simulink model "benchlink"  (R2024b)
settings: Solver=FixedStepDiscrete  StartTime=0.0  StopTime=0.005*16  RelTol=1e-3
model workspace (MAT data in the model file):
  socvcb : containers.Map (value not decoded)
values from neighbouring files (symbols this model uses):
  access = [32 0 4 36 32 0 4 36 32 0 4 36 ... (16 elements, 16x1)]    [all_variables.mat]
  qam_params =     [all_variables.mat]
undefined symbols (not defined in the file or in its folder): Add, j, QAM, rms, Shift
libraries: hdlsllib x53, simulink_need_slupdate x22, simulink x18, dspsigops x16, commdigbbndam3 x6, dsphdlmathfun2 x2, commchan3 x1, commrflib2 x1, dsphdlsigops2 x1, dspstat3 x1, dsphdlfiltering2 x1, simulink_extras x1
(part 5 of 5)

== matlab function benchlink/HDL_64QAM/HDLRxIPCore/QAM Rx HDL/Payload Delimiter/MATLAB Function1 ==
  data: isValid output; enable input; count input; isAccess output; qam_params parameter; accessChipStart input; packetSymLen input
function [isValid, isAccess] = ChipSync(enable, count, qam_params, accessChipStart, packetSymLen)
%#codegen

persistent state;
persistent counter;
%persistent packetLenInChips; % Renamed for clarity
persistent accessLen;

if isempty(state)
    state = false;
    counter = uint16(0);
    accessLen = uint16(qam_params.longTrainingChipLength);
end


packetLenInChips = uint16(packetSymLen * qam_params.spreadingFactor); 
isCountInRange = (mod(count, accessChipStart) < accessLen);


isCounterValid = (counter <= packetLenInChips) && (counter ~= 0);


isAccess = isCountInRange && isCounterValid;

if (counter <= packetLenInChips) && (counter ~= 0)
    isValid = true;
else
    isValid = false;
end
%%%%%%%%%%%%%%%%%%%%

% Internal logic using 'dvalid' (not an output) and decrementing counter
if state == false
    dvalid = false; % Not used as output
else % state == true
    dvalid = true;  % Not used as output
    % Decrement counter only when state is true
    if counter > 0
        counter = counter - 1;
    end
end

% state transition logic
if state == false && enable == true
    % Transition from false to true when enabled
    state = true;
    counter = packetLenInChips; % Use the pre-calculated value
elseif state == true && counter == 0
    % When state is true and counter reaches zero
    if enable == true
        % If still enabled, stay true and reset counter
        state = true;
        counter = packetLenInChips; % Use the pre-calculated value
    else
        % If not enabled when counter hits zero, transition back to false
        state = false;
        % Counter remains 0 until next enable
    end
end
% Implicit cases remain the same

end % End of function ChipSync

== matlab function benchlink/HDL_64QAM/HDLRxIPCore/QAM Rx HDL/EB Downsampler by 6_Old2/Chip Synchronization ==
  data: offset1 input; portSelect output; offset2 input; offset3 input; offset4 input; offset5 input; offset6 input
function portSelect  = chipSync(offset1, offset2, offset3, offset4, offset5, offset6)

[~,y] = max([offset1, offset2, offset3, offset4, offset5, offset6]);
portSelect = uint8(y);

== matlab function benchlink/HDL_64QAM/HDLRxIPCore/QAM Rx HDL/Payload Delimiter/Normalized Modulus/KeepMax ==
  data: in input; out output; qam_params parameter
function out  = keepMax(in, qam_params)

persistent x counter frameLen

if isempty(x)
    x = fi(0,1,18,15);
    counter    = uint16(0);
    frameLen = uint16((qam_params.packetSymLength*qam_params.spreadingFactor+...
        qam_params.preambleSymLength)*qam_params.Upsampling);
end

if (counter ~= 0)
    x = max(x,in);
    out = fi(x,1,18,15);
    counter = counter - 1;
else
    if (x > 5*in)
         out = fi(x,1,18,15);
         counter = frameLen;
    else
        x = fi(in,1,18,15);
        out = fi(x,1,18,15);
        counter = frameLen;
    end
end

== matlab function benchlink/HDL_64QAM/HDLRxIPCore/QAM Rx HDL/MF Filtering and Despreading/BER/ Integrate and Dump ==
  data: dValid input; validOut output; symbolIn input; sumOut output
function [validOut, sumOut] = intDump(dValid, symbolIn)
%#codegen

persistent sum_so_far counter

sumOut = fi(complex(0,0),1,18,13);
if isempty(sum_so_far)
sum_so_far = fi(complex(0,0),1,18,13);
end
validOut = false;
if isempty(counter)
counter = uint8(0);
end

if dValid
sum_so_far = fi(sum([sum_so_far symbolIn]),1,18,13);
counter = counter + 1;
end

if counter == 8
    sumOut = sum_so_far;
    validOut = true;
    counter = uint8(0);
    sum_so_far = fi(complex(0,0),1,18,13);
end

end

== matlab function benchlink/HDL_64QAM/HDLRxIPCore/QAM Rx HDL/MF Filtering and Despreading/BER/ Integrate and Dump1 ==
  data: dValid input; validOut output; symbolIn input; sumOut output
function [validOut, sumOut] = intDump(dValid, symbolIn)
%#codegen

persistent sum_so_far counter

sumOut = fi(complex(0,0),1,18,13);
if isempty(sum_so_far)
sum_so_far = fi(complex(0,0),1,18,13);
end
validOut = false;
if isempty(counter)
counter = uint8(0);
end

if dValid
sum_so_far = fi(sum([sum_so_far symbolIn]),1,18,13);
counter = counter + 1;
end

if counter == 8
    sumOut = sum_so_far;
    validOut = true;
    counter = uint8(0);
    sum_so_far = fi(complex(0,0),1,18,13);
end

end

== matlab function benchlink/HDL_64QAM/HDLRxIPCore/QAM Rx HDL/MF Filtering and Despreading/BER/BER Avg/MATLAB Function1 ==
  data: BERIn input; BERSumOut output; enable input; vecFullOut output; countOut output
function [BERSumOut, vecFullOut, countOut] = avgcodeVec(BERIn,enable)

persistent counter currVec fullVec isVecFull 

avgFactor = 8;

if isempty(counter)
    counter = uint8(0);
    currVec = ufi(0,19,9);
    fullVec = ufi(zeros(avgFactor,1),19,9);
    isVecFull = false;
end

if enable
    counter = counter + 1;
    fullVec(counter,:) = ufi(BERIn,19,9);
    if ~isVecFull
    currVec = ufi((currVec + BERIn),19,9);
    end
end

if isVecFull
    BERSumOut = ufi(sum(fullVec),19,9);
else
    BERSumOut = currVec;
end
countOut = counter;

if (counter == avgFactor)
        isVecFull = true;
        counter = uint8(0);
end
    
vecFullOut = isVecFull;

== matlab function benchlink/HDL_64QAM/HDLTxIPCore/QAMTxHDL/Controller FSM1 ==
  data: valid output; reset_preamble output; load_preamble output; load_data output; transmitNow input; packetsPerBurst input
function [valid, reset_preamble, load_preamble, load_data] = ControllerFSM(transmitNow,packetsPerBurst)
%#codegen
persistent packState stateCounter subDivCounter EoF txRequest 
%persistent packsIterate;
sType = numerictype(0,2,0);
cType = numerictype(0,16,0);
subDivType = numerictype(0,3,0); % Enough to count 0-7 for subdivisions

if isempty(packState)
    packState = fi(2,'numerictype',sType);
    stateCounter = fi(0,'numerictype',cType);
    subDivCounter = fi(0, 'numerictype', subDivType); % Initialize subdivision counter
    %packsIterate = uint16(packetsPerBurst - 1);
    EoF = true;
    txRequest = false;
end
Pack_Preamble = fi(0,'numerictype',sType);
Append_Data = fi(1,'numerictype',sType);

if transmitNow
    txRequest(:) = 1;
end

switch(packState)
    case Pack_Preamble
        % Pack_Preamble state handling code remains the same
        load_preamble = true;
        reset_preamble = false;
        load_data = false;
        valid = true;
        if stateCounter == uint16(31)
            packState(:) = 1;
            stateCounter(:) = 0;
            subDivCounter(:) = 0; % Ensure subdivision counter is reset here as well
        else
            stateCounter(:) = stateCounter + 1;
        end
    case Append_Data
        load_preamble = false;
        reset_preamble = true;
        load_data = true;
        valid = true;        
        if stateCounter == uint16(255)
            if subDivCounter == uint16(packetsPerBurst-1)
                packState(:) = 2;
                stateCounter(:) = 0;
                subDivCounter(:) = 0;
                EoF(:) = true;
                txRequest(:) = 0;
            else
                subDivCounter(:) = subDivCounter + 1;
                stateCounter(:) = 0; % Reset for next subdivision
            end
        else
            stateCounter(:) = stateCounter + 1;
        end
    otherwise
        load_preamble = false;
        reset_preamble = false;
        load_data = false;
        valid = false;
        if (txRequest && EoF)
            packState(:) = 0; % Reset to initial state if transmission request is active and EoF is true
        end
end% Assign the current value of stateCounter to the output variable for external use
%stateCounterOut = stateCounter;
end

== matlab function benchlink/HDL_64QAM/HDLRxIPCore/QAM Rx HDL/MF Filtering and Despreading/BER/BER Avg/MATLAB Function2 ==
  data: codeVec input; codeVecOut output; enable input; fullVecOut output; countOut output
function [codeVecOut, fullVecOut, countOut] = avgcodeVec(codeVec,enable)

persistent counter currVec fullVec

if isempty(counter)
    counter = uint8(0);
    currVec = sfi(0,19,9);
    fullVec = false;
end

if enable
    counter = counter + 1;
    currVec = sfi((currVec + codeVec),19,9);
end

codeVecOut = currVec;
countOut = counter;

if (counter == 8)
        fullVec = true;
        counter = uint8(0);
end
    
fullVecOut = fullVec;

== matlab function benchlink/HDL_64QAM/HDLRxIPCore/QAM Rx HDL/MF Filtering and Despreading/SymEVM/ Integrate and Dump ==
  data: dValid input; validOut output; symbolIn input; sumOut output
function [validOut, sumOut] = intDump(dValid, symbolIn)
%#codegen

persistent sum_so_far counter

sumOut = fi(complex(0,0),1,18,13);
if isempty(sum_so_far)
sum_so_far = fi(complex(0,0),1,18,13);
end
validOut = false;
if isempty(counter)
counter = uint8(0);
end

if dValid
sum_so_far = fi(sum([sum_so_far symbolIn]),1,18,13);
counter = counter + 1;
end

if counter == 8
    sumOut = sum_so_far;
    validOut = true;
    counter = uint8(0);
    sum_so_far = fi(complex(0,0),1,18,13);
end

end

== matlab function benchlink/HDL_64QAM/HDLTxIPCore/QAMTxHDL/Async FIFO/burstControl ==
  data: burstSize output; packetsPerBurst input; access_per_burst input
function burstSize  = burstControl(packetsPerBurst, access_per_burst)
    %#codegen    % Output logic based on the control input value
    if packetsPerBurst == 8 && access_per_burst == 1
        burstSize = uint16(1920);
    elseif packetsPerBurst == 8 && access_per_burst == 2
        burstSize = uint16(1792);
    elseif packetsPerBurst == 8 && access_per_burst == 4
        burstSize = uint16(1536);
    elseif packetsPerBurst == 8 && access_per_burst == 8
        burstSize = uint16(1024);
    elseif packetsPerBurst == 8 && access_per_burst == 6
        burstSize = uint16(1280);
    elseif packetsPerBurst == 4 && access_per_burst == 1
        burstSize = uint16(960);
    elseif packetsPerBurst == 4 && access_per_burst == 2
        burstSize = uint16(896);
    elseif packetsPerBurst == 4 && access_per_burst == 4
        burstSize = uint16(768);
    elseif packetsPerBurst == 2 && access_per_burst == 1
        burstSize = uint16(480);
    elseif packetsPerBurst == 2 && access_per_burst == 2
        burstSize = uint16(448);
    elseif packetsPerBurst == 2 && access_per_burst == 4
        burstSize = uint16(384);
    else
        burstSize = uint16(1920);
    end
end

== matlab function benchlink/HDL_64QAM/HDLRxIPCore/QAM Rx HDL/Payload Delimiter/MATLAB Function2 ==
  data: isValid output; enable input; count input; isAccess output; qam_params parameter; accessChipStart input; packetSymLen input
function [isValid,isAccess] = ChipSync(enable,count,qam_params,accessChipStart,packetSymLen)
%#codegen

persistent state;
persistent counter;
%persistent packetLen;
persistent accessLen; % Seems unused based on provided code
%persistent accessChipStart;

if isempty(state)
    state      = false;
    counter    = uint16(0);
    % Calculate packetLen based on qam_params
    %packetLen = uint16(packetSymLen * qam_params.spreadingFactor);
    accessLen = uint16(qam_params.longTrainingChipLength); % Initialize if needed
    %accessChipStart = uint32(qam_params.accessChipStart);
end


% Check if the input 'count' falls within the first 128 chips (0-127)
% of any 512-chip block within the 0-2047 range.
isCountInRange = (mod(count, accessChipStart) < accessLen);

% isValid is true when the internal counter is within the packet length and not zero.
isCounterValid = (counter <= (packetSymLen * qam_params.spreadingFactor)) && (counter ~= 0);

% Combine the conditions: isAccess is true only if the input 'count'
% is in a pilot range AND the internal counter state is valid.
isAccess = isCountInRange && isCounterValid;



if (counter <= (packetSymLen * qam_params.spreadingFactor)) && (counter ~= 0)
    isValid = true; % Renamed for clarity in comments: isInternalCounterActive = true;
else
    isValid = false; % Renamed for clarity in comments: isInternalCounterActive = false;
end
%%%%%%%%%%%%%%%%%%%%

% Internal logic using 'dvalid' (not an output) and decrementing counter
if state==false
    dvalid=false; % Not used as output
else %state==true
    dvalid=true;  % Not used as output
    % Decrement counter only when state is true (i.e., after being enabled
    % and before counting down to zero)
    if counter > 0 % Avoid decrementing when counter is already 0 before transition check
       counter = counter - 1;
    end
end

% state transition logic
if state==false && enable==true
    % Transition from false to true when enabled
    state=true;
    counter=packetSymLen * qam_params.spreadingFactor; % Reset/Load counter
elseif state==true && counter==0
    % When state is true and counter reaches zero (end of a packet count)
    if enable==true
        % If still enabled, stay true and reset counter (start next cycle)
        state      = true;
        counter    = packetSymLen * qam_params.spreadingFactor;
    else
        % If not enabled when counter hits zero, transition back to false
        state = false;
        % Counter remains 0 until next enable
    end
end
% Implicit cases:
% - If state is true and counter > 0, counter is decremented above.
% - If state is false and enable is false, nothing changes.

end % End of function ChipSync

== matlab function benchlink/HDL_64QAM/HDLRxIPCore/QAM Rx HDL/Payload Delimiter/ffcControl ==
  data: accessChipStart output; correctionsPerPack input
function accessChipStart  = ffcControl(correctionsPerPack)



    %#codegen    % Output logic based on the control input value
    if correctionsPerPack == 8
        accessChipStart = uint32(256);
    elseif correctionsPerPack == 4
        accessChipStart = uint32(512);
    elseif  correctionsPerPack == 2
        accessChipStart = uint32(1024);
    elseif correctionsPerPack == 1
        accessChipStart = uint32(2048);
    else
        accessChipStart = uint32(2048);
    end
end

== matlab function benchlink/HDL_64QAM/HDLRxIPCore/QAM Rx HDL/EB Downsampler by 6_old/Chip Synchronization ==
  data: offset1 input; portSelect output; offset2 input; offset3 input; offset4 input; offset5 input; offset6 input
function portSelect  = chipSync(offset1, offset2, offset3, offset4, offset5, offset6)

[~,y] = max([offset1, offset2, offset3, offset4, offset5, offset6]);
portSelect = uint8(y);

== matlab function benchlink/HDL_64QAM/HDLRxIPCore/QAM Rx HDL/Payload Delimiter/Normalized Modulus/KeepMaxSmallBurst ==
  data: in input; out output; qam_params parameter
function out  = keepMax(in, qam_params)

persistent x counter frameLen

if isempty(x)
    x = fi(0,1,18,15);
    counter    = uint16(0);
    frameLen = uint16((qam_params.packetSymLengthBig*qam_params.spreadingFactor+...
        qam_params.preambleSymLength)*qam_params.Upsampling);
end

if (counter ~= 0)
    x = max(x,in);
    out = fi(x,1,18,15);
    counter = counter - 1;
else
    if (x > 5*in)
         out = fi(x,1,18,15);
         counter = frameLen;
    else
        x = fi(in,1,18,15);
        out = fi(x,1,18,15);
        counter = frameLen;
    end
end

== matlab function benchlink/HDL_64QAM/HDLTxIPCore/QAMTxHDL/Async FIFO/burstControl2 ==
  data: output output; count input; num_blocks input
function output = processCountGeneral(count, num_blocks)
%#codegen
% Processes count based on equally spaced blocks (0-255 range).
% Assumes count is uint8 and num_blocks is a power of 2 (e.g., 2, 4)
% that divides 256. Outputs uint8.
% If count falls in the first 16 positions of a block, outputs the
% position (0-15), otherwise outputs 0.

    % Ensure coder directives for input types if not defined externally
    coder.allowpcode('plain'); % Standard directive for codegen
    % Assert input types (optional but good practice for clarity)
    % assert(isa(count, 'uint8'), 'Input count must be uint8');
    % assert(isa(num_blocks, 'uint8') || isa(num_blocks, 'uint16'), 'Input num_blocks must be an integer'); % Adjust type as needed

    % Define constants with explicit types (assuming uint16 for intermediate calculations)
    total_range_size = uint16(256);
    window_size      = uint16(16);
    num_blocks_u16   = uint16(num_blocks); % Cast num_blocks for calculations
    count_u16        = uint16(count);      % Cast count for calculations

    % --- Calculate block spacing using integer division ---
    % Use idivide for safe integer division. 'floor' is typical.
    % Ensure the divisor is also uint16.
    block_spacing = idivide(total_range_size, num_blocks_u16, 'floor'); % Result is uint16

    % --- Calculate position within the block using modulo ---
    % Both inputs to mod are now uint16
    position_in_block = mod(count_u16, block_spacing); % Result is uint16 (will be 0 to block_spacing-1)

    % --- Check if the position is within the pass-through window ---
    % Compare position_in_block (uint16) with window_size (uint16)
    if position_in_block < window_size
        % If yes, output the position within the window (0-15), cast to uint8
        output = uint8(position_in_block); % MODIFIED LINE
    else
        % If no, output zero, explicitly cast to the output type (uint8)
        output = uint8(0);
    end

end

== matlab function benchlink/HDL_64QAM/HDLTxIPCore/QAMTxHDL/Async FIFO/burstControl3 ==
  data: output output; count input; num_blocks input
function output = predictInverseWindow(count, num_blocks)
%#codegen
% Predicts if the *next* count value will fall outside the 0-15 window
% of its respective block within the 0-255 range.
% Assumes count is uint8 and num_blocks is a power of 2 (e.g., 1, 2, 4)
% that divides 256. Outputs uint8 (1 or 0).
%
% Output is 1 if (count+1) is NOT in a 0-15 window.
% Output is 0 if (count+1) IS in a 0-15 window.

    % Ensure coder directives for input types if not defined externally
    coder.allowpcode('plain'); % Standard directive for codegen

    % Define constants with explicit types (using uint16 for safety)
    total_range_size = uint16(256);
    window_size      = uint16(16);
    num_blocks_u16   = uint16(num_blocks); % Cast num_blocks
    count_u16        = uint16(count);      % Cast current count

    % --- Calculate the next count value (handles wrap-around via modulo later) ---
    % We need to check the state for 'count + 1'
    next_count_u16 = count_u16 + 1;
    % Note: If count is 255, next_count_u16 becomes 256.

    % --- Calculate block spacing using integer division ---
    % Assuming num_blocks is valid (positive, divides 256) for HDL
    block_spacing = idivide(total_range_size, num_blocks_u16, 'floor'); % Result is uint16

    % --- Calculate position of the *next* count within its block ---
    % Modulo handles the wrap-around: mod(256, block_spacing) will be 0.
    next_position_in_block = mod(next_count_u16, block_spacing); % Result is uint16

    % --- Check if the *next* position falls within the 0-15 window ---
    if next_position_in_block < window_size
        % If next count IS in a window, output 0 for the current count
        output = uint8(0);
    else
        % If next count is NOT in a window, output 1 for the current count
        output = uint8(1);
    end

end

== matlab function benchlink/HDL_64QAM/HDLTxIPCore/QAMTxHDL/Async FIFO/burstControl4 ==
  data: output output; count input; num_blocks input
function output = isInWindow(count, num_blocks)
%#codegen
% Checks if the current count falls within the 0-15 window of its
% respective block within the 0-255 range.
% Assumes count is uint8 and num_blocks is a power of 2 (e.g., 1, 2, 4)
% that divides 256. Outputs uint8 (1 or 0).
%
% Output is 1 if count IS in a 0-15 window.
% Output is 0 if count is NOT in a 0-15 window.

    % Ensure coder directives for input types if not defined externally
    coder.allowpcode('plain'); % Standard directive for codegen

    % Define constants with explicit types (using uint16 for safety)
    total_range_size = uint16(256);
    window_size      = uint16(16);
    num_blocks_u16   = uint16(num_blocks); % Cast num_blocks
    count_u16        = uint16(count);      % Cast current count

    % --- Calculate block spacing using integer division ---
    % Assuming num_blocks is valid (positive, divides 256) for HDL
    block_spacing = idivide(total_range_size, num_blocks_u16, 'floor'); % Result is uint16

    % --- Calculate position of the *current* count within its block ---
    position_in_block = mod(count_u16, block_spacing); % Result is uint16

    % --- Check if the *current* position falls within the 0-15 window ---
    if position_in_block < window_size
        % If current count IS in a window, output 1
        output = uint8(1);
    else
        % If current count is NOT in a window, output 0
        output = uint8(0);
    end

end
